simulink model "Model_7ent2062_2026"  (R2025b)
settings: Solver=ode1  StartTime=0  StopTime=Tend  FixedStep=0.1  RelTol=1e-3
values from neighbouring files (symbols this model uses):
  regenRate = 0.25    [Script_7ent1162_2026.m]
undefined symbols (not defined in the file or in its folder): battery, coef, Ion, Lithium, vehicle
libraries: autolibshared x1, spsBatteryLib x1, simulink x1, spsControlledCurrentSourceLib x1, spspowerguiLib x1
settings Model: Creator=kl20aah  LastModifiedBy=Rupeshwaran
settings DataIOCC: SaveFormat=StructureWithTime  SaveOutput=off  SignalLogging=off  DSMLogging=off  ReturnWorkspaceOutputs=off
settings RTWCC: GPUComputeCapability=3.5

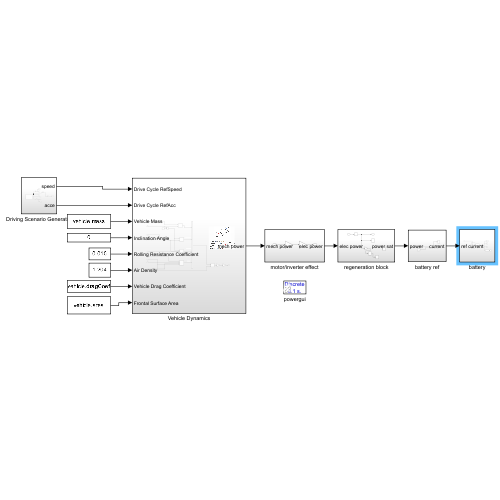
[thumbnail: Simulink's stored preview of the top-level diagram]
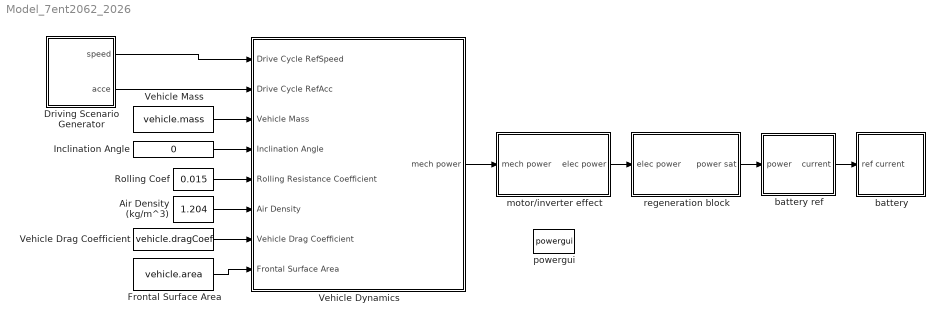
== system Model_7ent2062_2026 ==
  Air Density (kg/m^3) : Constant  Value=1.204
  Driving Scenario Generator : Subsystem
  Frontal Surface Area : Constant  Value=vehicle.area
  Inclination Angle : Constant  Value=0
  Rolling Coef : Constant  Value=0.015
  Vehicle Drag Coefficient : Constant  Value=vehicle.dragCoef
  Vehicle Dynamics : Subsystem
  Vehicle Mass : Constant  Value=vehicle.mass
  battery : Subsystem
  battery ref : Subsystem
  motor/inverter effect : Subsystem
  powergui : spspowerguiLib/powergui  Priority=1  SimulationMode=Discrete  SampleTime=0.1  frequency=60  Iterations=50  frequencyindice=0  Pbase=100e6  ErrMax=1e-4  UnitsV=kV  UnitsW=MW  buscounter=0  FunctionMessages=off  echomessages=off  EnableUseOfTLC=off  CurrentSourceSwitches=off  DisableSnubberDevices=off  DisableRonSwitches=off  DisableVfSwitches=off  DisplayEquations=off  AutomaticDiscreteSolvers=off  SolverType=Tustin/Backward Euler (TBE)  Interpol=off  ExternalGateDelay=off  methode=off  Ts=100  x0status=blocks  SPID=on  SwTol=0  HookPort=off  NonlinearTolerance=1e-4  nMaxIteration=100  ContinueOnMaxIteration=off  RestoreLinks=warning  ResistiveCurrentMeasurement=off  Frange=[0:2:500]  Ylog=off  Xlog=on  ShowGrid=off  save=off  variable=ZData  structure=0  ZoomFFT=off  StartTime=0.0  cycles=1  DisplayStyle=1  fundamental=60  FreqAxis=off  MaxFrequency=1000  frequencyindicesteady=1  RmsSteady=1  display=off
  regeneration block : Subsystem
  wires:
  Driving Scenario Generator/1(speed) -> Vehicle Dynamics/1(Drive Cycle RefSpeed)
  Driving Scenario Generator/2(acce) -> Vehicle Dynamics/2(Drive Cycle RefAcc)
  Vehicle Mass/1 -> Vehicle Dynamics/3(Vehicle Mass)
  Inclination Angle/1 -> Vehicle Dynamics/4(Inclination Angle)
  Rolling Coef/1 -> Vehicle Dynamics/5(Rolling Resistance Coefficient)
  Air Density (kg/m^3)/1 -> Vehicle Dynamics/6(Air Density)
  Vehicle Drag Coefficient/1 -> Vehicle Dynamics/7(Vehicle Drag Coefficient)
  Frontal Surface Area/1 -> Vehicle Dynamics/8(Frontal Surface Area)
  Vehicle Dynamics/1(mech power) -> motor/inverter effect/1(mech power)
  motor/inverter effect/1(elec power) -> regeneration block/1(elec power)
  regeneration block/1(power sat) -> battery ref/1(power)
  battery ref/1(current) -> battery/1(ref current)

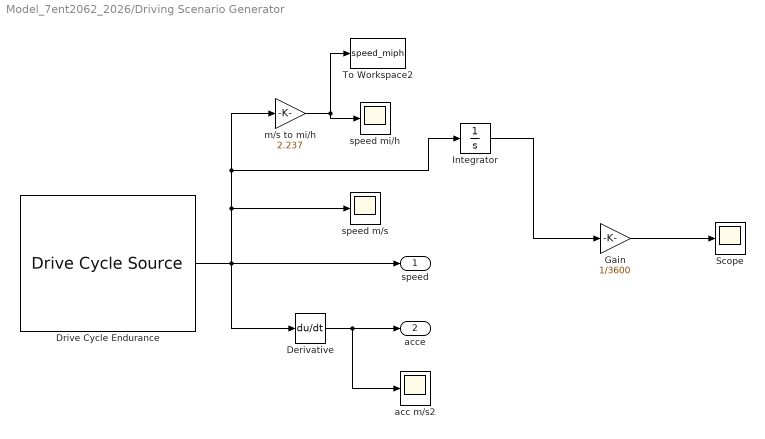
== system Model_7ent2062_2026/Driving Scenario Generator ==
  Derivative : Derivative
  Drive Cycle Endurance : autolibshared/Drive Cycle Source  cycleVar=Workspace variable  wsVar=myCycle  fileVar=cycleFTP75.mat  tfinal="993  seconds, Cyclic"  cycleRepeat=on  outAccPort=off  outGearPort=off  gearList=No gear data  t_wot1=5  xdot_woto=0  xdot_wot1=30  t_wot2=20  xdot_wot2=0  t_wotend=30  srcUnit=m/s  outUnit=m/s  srcAccUnit=m/s/s  outAccUnit=m/s^2  dt=0.1  aMode=1  faultOption=off  velBnd=2  velBndUnit=mph  inUnit=m/s  timeBnd=1  failOption=off  stopSim=off  maxFaultCnt=10  maxFaultTime=2  maxTotFaultTime=15  traceOption=off  dtTrace=1  traceWindow=10  lastDCname=Custom Data Set  lastOutUnit=mph  lastDT=0.1  lastTB=1  lastSB=2  forceCalcBound=off
  Gain : Gain  Gain=1/3600
  Integrator : Integrator
  Scope : Scope
      settings: Title=Drive cycle 1  ActiveDisplayYMinimum=-93.429702835676451  ActiveDisplayYMaximum=840.86732552108822  YLabel=Distance travel  DataLoggingVariableName=ScopeData4
  To Workspace2 : ToWorkspace  VariableName=speed_miph  SampleTime=-1
      settings: Save2DSignal=2-D array (concatenate along first dimension)
  acc m/s2 : Scope
      settings: ActiveDisplayYMinimum=-1.90625  ActiveDisplayYMaximum=2.15625  DataLoggingVariableName=ScopeData3
  m/s to mi/h : Gain  Gain=2.237
  speed m/s : Scope
      settings: ActiveDisplayYMinimum=-1.41935  ActiveDisplayYMaximum=12.77417
  speed mi/h : Scope
      settings: ActiveDisplayYMinimum=-10.19855  ActiveDisplayYMaximum=91.78691  DataLoggingVariableName=ScopeData2
  speed : Outport
  acce : Outport  Port=2
  wires:
  m/s to mi/h/1 -> To Workspace2/1, speed mi/h/1
  Drive Cycle Endurance/1 -> m/s to mi/h/1, Integrator/1, speed m/s/1, Derivative/1, speed/1
  Derivative/1 -> acc m/s2/1, acce/1
  Integrator/1 -> Gain/1
  Gain/1 -> Scope/1

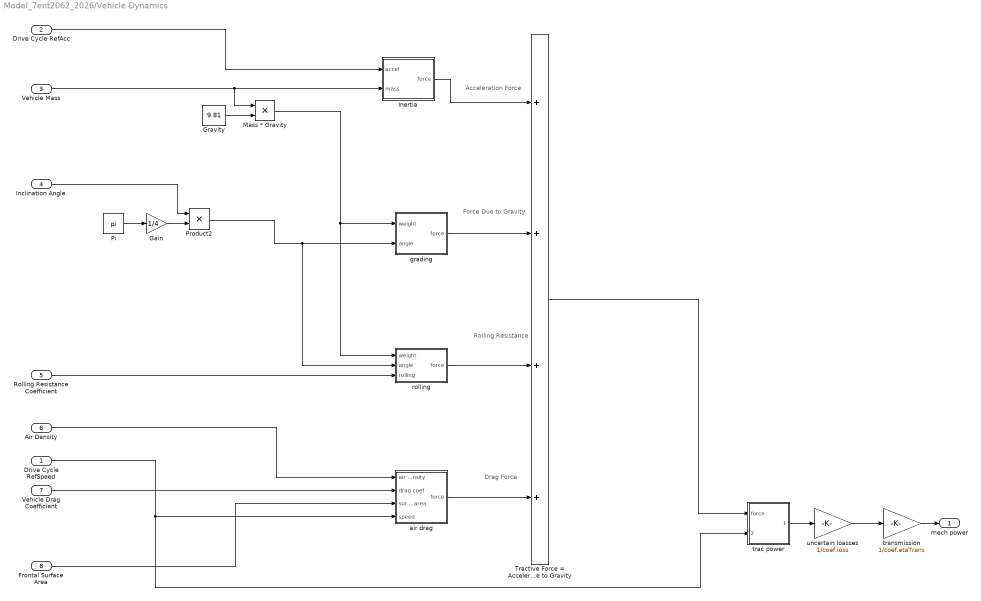
== system Model_7ent2062_2026/Vehicle Dynamics ==
  note: Drag Force
  note: Rolling Resistance
  note: Force Due to Gravity
  note: Acceleration Force
  Drive Cycle RefSpeed : Inport
  Drive Cycle RefAcc : Inport  Port=2
  Vehicle Mass : Inport  Port=3
  Inclination Angle : Inport  Port=4
  Rolling Resistance Coefficient : Inport  Port=5
  Air Density : Inport  Port=6
  Vehicle Drag Coefficient : Inport  Port=7
  Frontal Surface Area : Inport  Port=8
  Gain : Gain  Gain=1/4
  Gravity : Constant  Value=9.81
  Inertia : Subsystem
  Mass * Gravity : Product
  Pi : Constant  Value=pi  OutDataTypeStr=Inherit: Inherit via back propagation
  Product2 : Product
  Tractive Force = Acceleration Force + Drag Force + Rolling Resistance + Force Due to Gravity : Sum  Inputs=++++
  air drag : Subsystem
  grading : Subsystem
  rolling : Subsystem
  trac power : Subsystem
  transmission : Gain  Gain=1/coef.etaTrans
  uncertain loasses : Gain  Gain=1/coef.loss
  mech power : Outport
  wires:
  Vehicle Mass/1 -> Inertia/2(mass), Mass * Gravity/1
  Inclination Angle/1 -> Product2/1
  Pi/1 -> Gain/1
  Gain/1 -> Product2/2
  Gravity/1 -> Mass * Gravity/2
  Inertia/1(force) -> Tractive Force = Acceleration Force + Drag Force + Rolling Resistance + Force Due to Gravity/1
  grading/1(force) -> Tractive Force = Acceleration Force + Drag Force + Rolling Resistance + Force Due to Gravity/2
  rolling/1(force) -> Tractive Force = Acceleration Force + Drag Force + Rolling Resistance + Force Due to Gravity/3
  air drag/1(force) -> Tractive Force = Acceleration Force + Drag Force + Rolling Resistance + Force Due to Gravity/4
  Drive Cycle RefAcc/1 -> Inertia/1(accel)
  Product2/1 -> rolling/2(angle), grading/2(angle)
  Mass * Gravity/1 -> rolling/1(weight), grading/1(weight)
  Rolling Resistance Coefficient/1 -> rolling/3(rolling)
  Frontal Surface Area/1 -> air drag/3(surface area)
  Vehicle Drag Coefficient/1 -> air drag/2(drag coef)
  Drive Cycle RefSpeed/1 -> trac power/2(speed), air drag/4(speed)
  Air Density/1 -> air drag/1(air density)
  Tractive Force = Acceleration Force + Drag Force + Rolling Resistance + Force Due to Gravity/1 -> trac power/1(force)
  trac power/1(power) -> uncertain loasses/1
  uncertain loasses/1 -> transmission/1
  transmission/1 -> mech power/1

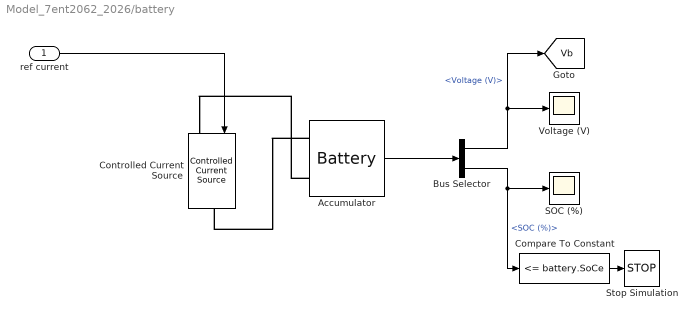
== system Model_7ent2062_2026/battery ==
  ref current : Inport
  Accumulator : spsBatteryLib/Battery  BatType=Lithium-Ion  NomV=battery.Vnom  NomQ=battery.AHrat  SOC=battery.SoCi  Batt_Tr=300  PresetModel=on  MaxQ=349.77  MinV=273.75  FullV=424.8553  Dis_rate=152.0739  R=0.010435  Normal_OP=316.3137  expZone="[394.3408      17.18435]"
  Bus Selector : BusSelector  OutputSignals=Voltage (V),SOC (%)
  Compare To Constant : simulink/Logic and Bit Operations/Compare To Constant  relop=<=  const=battery.SoCe  OutDataTypeStr=boolean
  Controlled Current Source : spsControlledCurrentSourceLib/Controlled Current Source  Initialize=on  Source_Type=DC  Amplitude=0  Phase=0  Frequency=0  Measurements=None
  SOC (%) : Scope
      settings: ActiveDisplayYMinimum=100.06698411473212  ActiveDisplayYMaximum=103.41234978160016  DataLoggingVariableName=ScopeData3
  Stop Simulation : Stop
  Voltage (V) : Scope
      settings: ActiveDisplayYMinimum=403.4768  ActiveDisplayYMaximum=448.77222  DataLoggingVariableName=ScopeData2
  tag scope: Vb=global
  wires:
  Bus Selector/2 -> Compare To Constant/1, SOC (%)/1  "<SOC (%)>"
  Compare To Constant/1 -> Stop Simulation/1
  Bus Selector/1 -> [Vb], Voltage (V)/1  "<Voltage (V)>"
  ref current/1 -> Controlled Current Source/1
  Accumulator/1 -> Bus Selector/1
  connections:
  Accumulator/LConn2 -- Controlled Current Source/RConn1
  Accumulator/LConn1 -- Controlled Current Source/LConn1

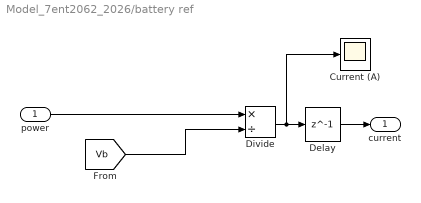
== system Model_7ent2062_2026/battery ref ==
  power : Inport
  Current (A) : Scope
      settings: ActiveDisplayYMinimum=-168.1133  ActiveDisplayYMaximum=258.01973
  Delay : Delay  DelayLength=1
  Divide : Product  Inputs=*/
  current : Outport
  wires:
  power/1 -> Divide/1
  [Vb] -> Divide/2
  Divide/1 -> Current (A)/1, Delay/1
  Delay/1 -> current/1

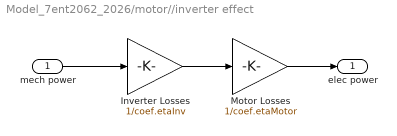
== system Model_7ent2062_2026/motor//inverter effect ==
  mech power : Inport
  Inverter Losses : Gain  Gain=1/coef.etaInv
  Motor Losses : Gain  Gain=1/coef.etaMotor
  elec power : Outport
  wires:
  Inverter Losses/1 -> Motor Losses/1
  Motor Losses/1 -> elec power/1
  mech power/1 -> Inverter Losses/1

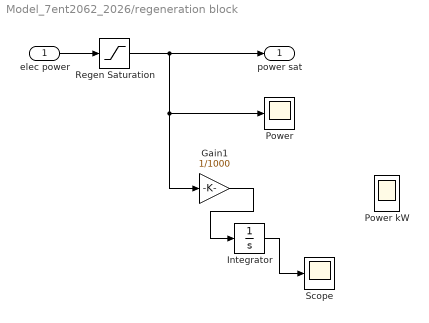
== system Model_7ent2062_2026/regeneration block ==
  elec power : Inport
  Gain1 : Gain  Gain=1/1000
  Integrator : Integrator
  Power : Scope
      settings: TimeSpan=993  Title=Drive cycle one  ActiveDisplayYMinimum=-31520.290121433281  ActiveDisplayYMaximum=97590.040267301025  YLabel=Electric power demand  DataLoggingVariableName=ScopeData6
  Power kW : Scope
      settings: TimeSpan=993  Title=Drive cycle 2  ActiveDisplayYMinimum=-105.05967635270716  ActiveDisplayYMaximum=115.70776217436436  YLabel=Electric power demand (Kw)  DataLoggingVariableName=ScopeData5
  Regen Saturation : Saturate  UpperLimit=inf  LowerLimit=-regenRate*(battery.Vnom*battery.AHrat)
  Scope : Scope
      settings: Title=DRIVE CYCLE 1  ActiveDisplayYMinimum=240053.05516635466  ActiveDisplayYMaximum=278676.2700578043  YLabel=Electric power demand (kW)  DataLoggingVariableName=ScopeData7
  power sat : Outport
  wires:
  Gain1/1 -> Integrator/1
  elec power/1 -> Regen Saturation/1
  Regen Saturation/1 -> Gain1/1, Power/1, power sat/1
  Integrator/1 -> Scope/1

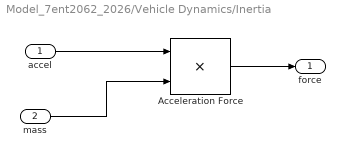
== system Model_7ent2062_2026/Vehicle Dynamics/Inertia ==
  accel : Inport
  mass : Inport  Port=2
  Acceleration Force : Product
  force : Outport
  wires:
  accel/1 -> Acceleration Force/1
  mass/1 -> Acceleration Force/2
  Acceleration Force/1 -> force/1

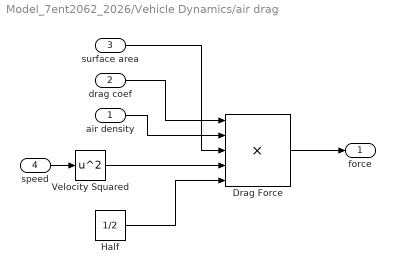
== system Model_7ent2062_2026/Vehicle Dynamics/air drag ==
  air density : Inport
  drag coef : Inport  Port=2
  surface area : Inport  Port=3
  speed : Inport  Port=4
  Drag Force : Product  Inputs=5
  Half : Constant  Value=1/2
  Velocity Squared : Math  Operator=square
  force : Outport
  wires:
  Drag Force/1 -> force/1
  Half/1 -> Drag Force/5
  drag coef/1 -> Drag Force/1
  air density/1 -> Drag Force/2
  speed/1 -> Velocity Squared/1
  Velocity Squared/1 -> Drag Force/4
  surface area/1 -> Drag Force/3

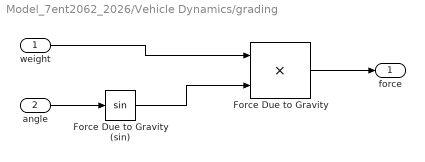
== system Model_7ent2062_2026/Vehicle Dynamics/grading ==
  weight : Inport
  angle : Inport  Port=2
  Force Due to Gravity : Product
  Force Due to Gravity (sin) : Trigonometry
  force : Outport
  wires:
  angle/1 -> Force Due to Gravity (sin)/1
  Force Due to Gravity (sin)/1 -> Force Due to Gravity/2
  weight/1 -> Force Due to Gravity/1
  Force Due to Gravity/1 -> force/1

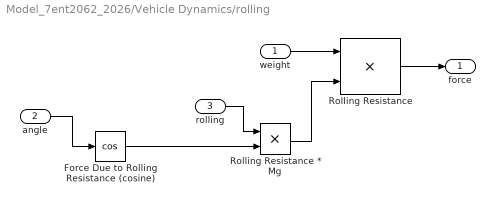
== system Model_7ent2062_2026/Vehicle Dynamics/rolling ==
  weight : Inport
  angle : Inport  Port=2
  rolling : Inport  Port=3
  Force Due to Rolling Resistance (cosine) : Trigonometry  Operator=cos
  Rolling Resistance : Product
  Rolling Resistance * Mg : Product
  force : Outport
  wires:
  Rolling Resistance/1 -> force/1
  angle/1 -> Force Due to Rolling Resistance (cosine)/1
  Force Due to Rolling Resistance (cosine)/1 -> Rolling Resistance * Mg/2
  rolling/1 -> Rolling Resistance * Mg/1
  Rolling Resistance * Mg/1 -> Rolling Resistance/2
  weight/1 -> Rolling Resistance/1

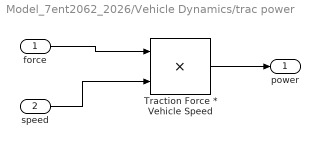
== system Model_7ent2062_2026/Vehicle Dynamics/trac power ==
  force : Inport
  speed : Inport  Port=2
  Traction Force * Vehicle Speed : Product
  power : Outport
  wires:
  Traction Force * Vehicle Speed/1 -> power/1
  speed/1 -> Traction Force * Vehicle Speed/2
  force/1 -> Traction Force * Vehicle Speed/1
